simulink model "train_model_la_nika"  (R2021b)
settings: Solver=VariableStepAuto  StartTime=0.0  StopTime=20  RelTol=1e-3
values from neighbouring files (symbols this model uses):
  g = 9.8    [sis_init.m]
  n_y = 1    [sis_init.m]
  n_z = 0    [sis_init.m]
  speed_tgt = 100    [sis_init.m]
  speed_tgt_2 = 130    [sis_init.m]
  v0 = 20    [sis_init.m]
settings Model: Creator=Acer  LastModifiedBy=Acer

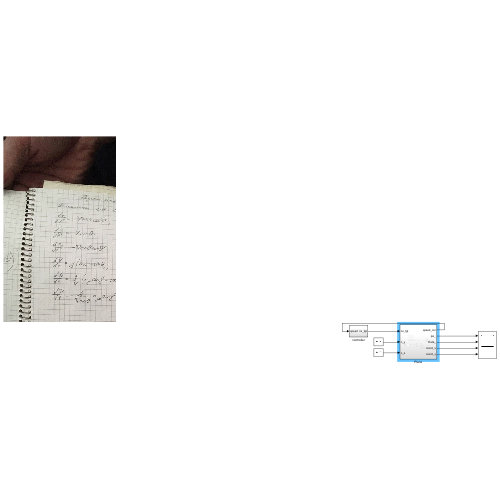
[thumbnail: Simulink's stored preview of the top-level diagram]
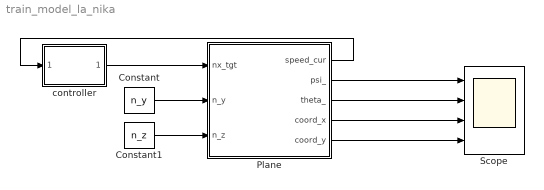
== system train_model_la_nika ==
  Constant : Constant  Value=n_y
  Constant1 : Constant  Value=n_z
  Plane : Subsystem
  Scope : Scope  NumInputPorts=4
  controller : Subsystem
  wires:
  Plane/1(speed_cur) -> controller/1(speed)
  controller/1(nx_tgt) -> Plane/1(nx_tgt)
  Constant/1 -> Plane/2(n_y)
  Constant1/1 -> Plane/3(n_z)
  Plane/4(coord_x) -> Scope/3
  Plane/5(coord_y) -> Scope/4
  Plane/3(theta_) -> Scope/2
  Plane/2(psi_) -> Scope/1

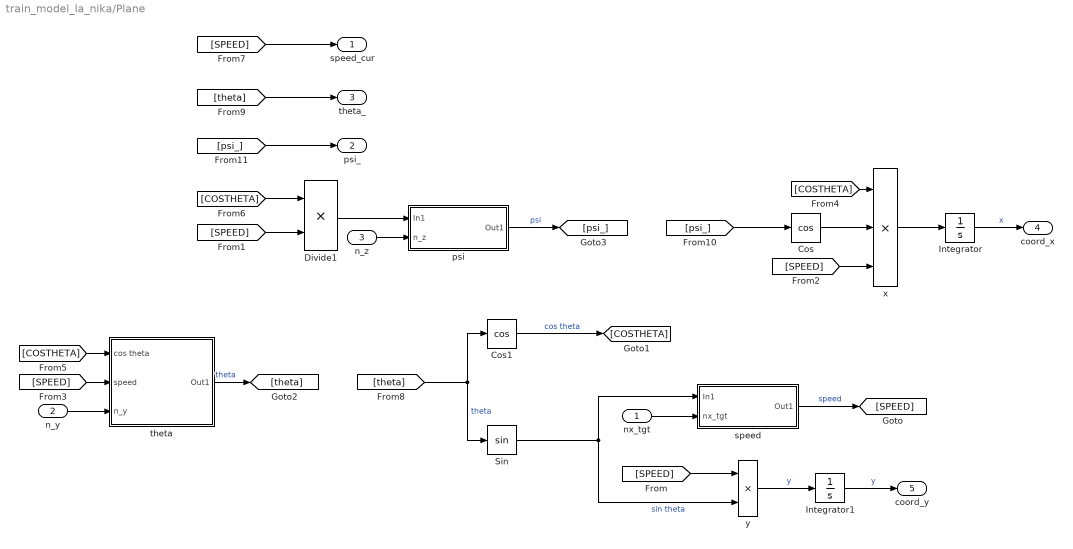
== system train_model_la_nika/Plane ==
  nx_tgt : Inport
  n_y : Inport  Port=2
  n_z : Inport  Port=3
  Cos : Trigonometry  Operator=cos
  Cos1 : Trigonometry  Operator=cos
  Divide1 : Product  Inputs=**
  Integrator : Integrator
  Integrator1 : Integrator  InitialCondition=1000  UpperSaturationLimit=1000
  Sin : Trigonometry
  psi : Subsystem
  speed : Subsystem
  theta : Subsystem
  x : Product  Inputs=***
  y : Product  Inputs=**
  speed_cur : Outport
  psi_ : Outport  Port=2
  theta_ : Outport  Port=3
  coord_x : Outport  Port=4
  coord_y : Outport  Port=5
  wires:
  [SPEED] -> y/1
  x/1 -> Integrator/1
  [COSTHETA] -> x/1
  [SPEED] -> theta/2(speed)
  [SPEED] -> Divide1/2
  y/1 -> Integrator1/1  "y"
  speed/1(Out1) -> [SPEED]  "speed"
  Sin/1 -> speed/1(In1), y/2  "sin theta"
  Divide1/1 -> psi/1(In1)
  [COSTHETA] -> Divide1/1
  [SPEED] -> x/3
  [COSTHETA] -> theta/1(cos theta)
  Cos1/1 -> [COSTHETA]  "cos theta"
  Cos/1 -> x/2
  [SPEED] -> speed_cur/1
  nx_tgt/1 -> speed/2(nx_tgt)
  n_y/1 -> theta/3(n_y)
  n_z/1 -> psi/2(n_z)
  Integrator/1 -> coord_x/1  "х"
  Integrator1/1 -> coord_y/1  "y"
  theta/1(Out1) -> [theta]  "theta"
  [theta] -> Sin/1, Cos1/1  "theta"
  [theta] -> theta_/1
  psi/1(Out1) -> [psi_]  "psi"
  [psi_] -> Cos/1
  [psi_] -> psi_/1

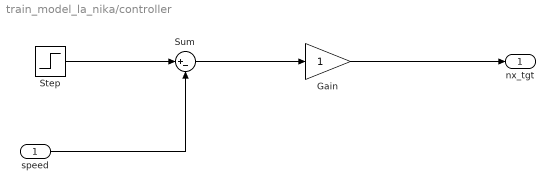
== system train_model_la_nika/controller ==
  speed : Inport
  Gain : Gain
  Step : Step  Time=10  Before=speed_tgt  After=speed_tgt_2  SampleTime=0
  Sum : Sum  Inputs=|+-
  nx_tgt : Outport
  wires:
  Sum/1 -> Gain/1
  Step/1 -> Sum/1
  Gain/1 -> nx_tgt/1
  speed/1 -> Sum/2

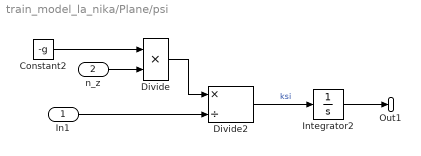
== system train_model_la_nika/Plane/psi ==
  In1 : Inport
  n_z : Inport  Port=2
  Constant2 : Constant  Value=-g
  Divide : Product  Inputs=**
  Divide2 : Product  Inputs=*/
  Integrator2 : Integrator
  Out1 : Outport
  wires:
  Divide2/1 -> Integrator2/1  "ksi"
  In1/1 -> Divide2/2
  Integrator2/1 -> Out1/1
  Constant2/1 -> Divide/1
  n_z/1 -> Divide/2
  Divide/1 -> Divide2/1

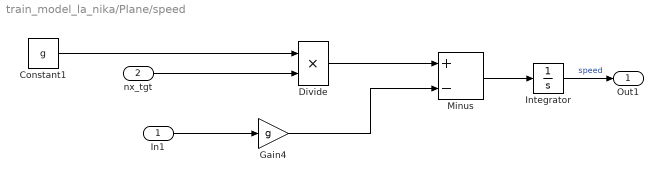
== system train_model_la_nika/Plane/speed ==
  In1 : Inport
  nx_tgt : Inport  Port=2
  Constant1 : Constant  Value=g
  Divide : Product  Inputs=**
  Gain4 : Gain  Gain=g
  Integrator : Integrator  InitialCondition=v0
  Minus : Sum  Inputs=+-
  Out1 : Outport
  wires:
  Minus/1 -> Integrator/1
  Gain4/1 -> Minus/2
  Integrator/1 -> Out1/1  "speed"
  In1/1 -> Gain4/1
  Constant1/1 -> Divide/1
  nx_tgt/1 -> Divide/2
  Divide/1 -> Minus/1

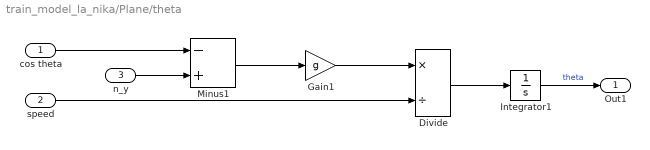
== system train_model_la_nika/Plane/theta ==
  cos theta : Inport
  speed : Inport  Port=2
  n_y : Inport  Port=3
  Divide : Product  Inputs=*/
  Gain1 : Gain  Gain=g
  Integrator1 : Integrator
  Minus1 : Sum  Inputs=-+
  Out1 : Outport
  wires:
  Gain1/1 -> Divide/1
  Minus1/1 -> Gain1/1
  n_y/1 -> Minus1/2
  Divide/1 -> Integrator1/1
  Integrator1/1 -> Out1/1  "theta"
  cos theta/1 -> Minus1/1
  speed/1 -> Divide/2
